simulink model "SinusAbsolueIntegree"  (R2016b)
settings: Solver=VariableStepAuto  StartTime=0.0  StopTime=10.0  RelTol=1e-3
settings Model: Creator=live  LastModifiedBy=live

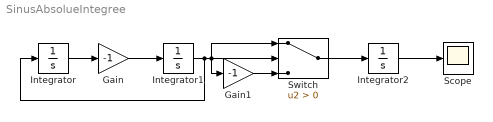
== system SinusAbsolueIntegree ==
  Gain : Gain  Gain=-1
  Gain1 : Gain  Gain=-1
  Integrator : Integrator  InitialCondition=1
  Integrator1 : Integrator
  Integrator2 : Integrator
  Scope : Scope
  Switch : Switch  Criteria=u2 > Threshold
  wires:
  Integrator/1 -> Gain/1
  Gain/1 -> Integrator1/1
  Integrator1/1 -> Integrator/1, Gain1/1, Switch/1, Switch/2
  Gain1/1 -> Switch/3
  Switch/1 -> Integrator2/1
  Integrator2/1 -> Scope/1
